simulink model "DDMRModel"  (R2023b)
settings: Solver=VariableStepAuto  StartTime=0.0  StopTime=3  RelTol=1e-3
undefined symbols (not defined in the file or in its folder): Bm, gR, Jm, Kd, ke, Ki, Kp, kt, L, La, R, Ra
settings Model: Creator=rodrigoscott  LastModifiedBy=rodrigoscott

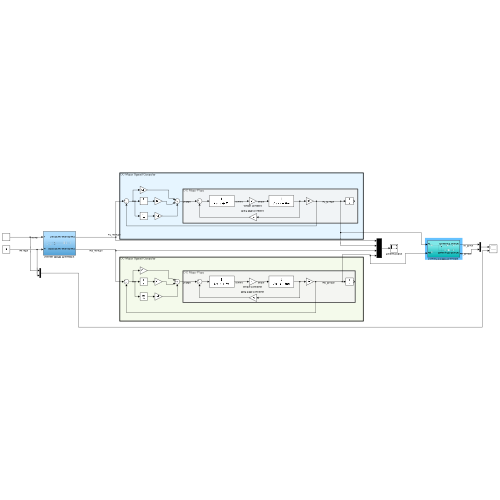
[thumbnail: Simulink's stored preview of the top-level diagram]
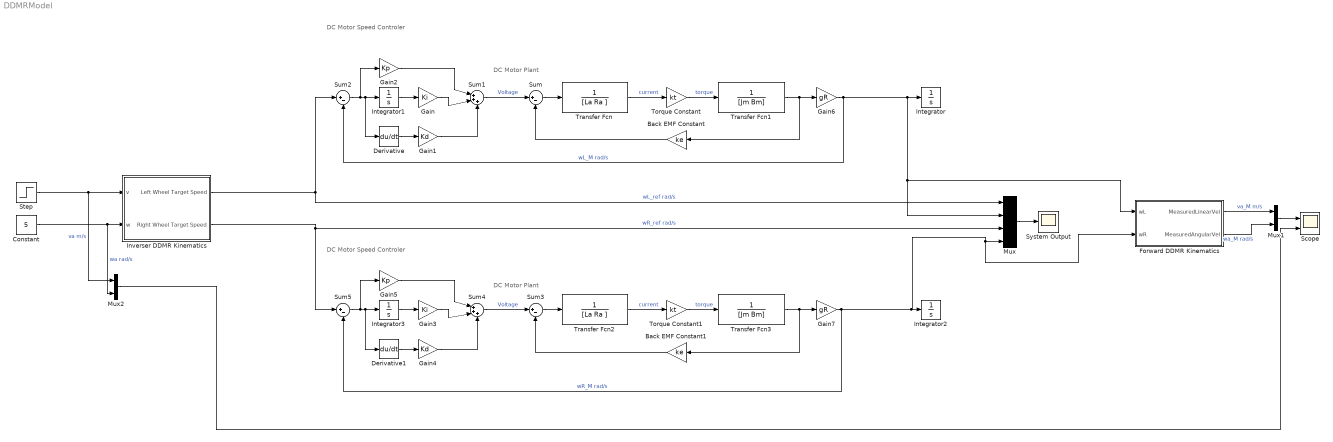
== system DDMRModel ==
  note: DC Motor Speed Controler
  note: DC Motor Plant
  note: DC Motor Plant
  note: DC Motor Speed Controler
  Back EMF Constant : Gain  Gain=ke
  Back EMF Constant1 : Gain  Gain=ke
  Constant : Constant  Value=5
  Derivative : Derivative
  Derivative1 : Derivative
  Forward DDMR Kinematics : Subsystem
  Gain : Gain  Gain=Ki
  Gain1 : Gain  Gain=Kd
  Gain2 : Gain  Gain=Kp
  Gain3 : Gain  Gain=Ki
  Gain4 : Gain  Gain=Kd
  Gain5 : Gain  Gain=Kp
  Gain6 : Gain  Gain=gR
  Gain7 : Gain  Gain=gR
  Integrator{,1..3} (4 alike) : Integrator
  Inverser DDMR Kinematics : Subsystem
  Mux : Mux
  Mux1 : Mux  Inputs=2
  Mux2 : Mux  Inputs=2
  Scope : Scope  NumInputPorts=2
  Step : Step  Time=0  SampleTime=0
  Sum{,2..3,5} (4 alike) : Sum  Inputs=|+-
  Sum1 : Sum  Inputs=|+++
  Sum4 : Sum  Inputs=|+++
  System Output : Scope
  Torque Constant : Gain  Gain=kt
  Torque Constant1 : Gain  Gain=kt
  Transfer Fcn : TransferFcn  Denominator=[La Ra ]
  Transfer Fcn1 : TransferFcn  Denominator=[Jm Bm]
  Transfer Fcn2 : TransferFcn  Denominator=[La Ra ]
  Transfer Fcn3 : TransferFcn  Denominator=[Jm Bm]
  wires:
  Sum1/1 -> Sum/1  "Voltage"
  Transfer Fcn/1 -> Torque Constant/1  "current"
  Sum/1 -> Transfer Fcn/1
  Transfer Fcn1/1 -> Back EMF Constant/1, Gain6/1
  Sum2/1 -> Gain2/1, Derivative/1, Integrator1/1
  Back EMF Constant/1 -> Sum/2
  Gain1/1 -> Sum1/3
  Torque Constant/1 -> Transfer Fcn1/1  "torque"
  Integrator1/1 -> Gain/1
  Gain/1 -> Sum1/2
  Gain2/1 -> Sum1/1
  Derivative/1 -> Gain1/1
  Transfer Fcn3/1 -> Back EMF Constant1/1, Gain7/1
  Back EMF Constant1/1 -> Sum3/2
  Transfer Fcn2/1 -> Torque Constant1/1  "current"
  Torque Constant1/1 -> Transfer Fcn3/1  "torque"
  Gain4/1 -> Sum4/3
  Sum3/1 -> Transfer Fcn2/1
  Sum5/1 -> Gain5/1, Derivative1/1, Integrator3/1
  Gain3/1 -> Sum4/2
  Gain5/1 -> Sum4/1
  Derivative1/1 -> Gain4/1
  Sum4/1 -> Sum3/1  "Voltage"
  Integrator3/1 -> Gain3/1
  Inverser DDMR Kinematics/1(Left Wheel Target Speed) -> Sum2/1, Mux/1  "wL_ref rad/s"
  Inverser DDMR Kinematics/2(Right Wheel Target Speed) -> Sum5/1, Mux/3  "wR_ref rad/s"
  Step/1 -> Mux2/1, Inverser DDMR Kinematics/1(v)  "va m/s"
  Constant/1 -> Mux2/2, Inverser DDMR Kinematics/2(w)  "wa rad/s"
  Gain6/1 -> Sum2/2, Integrator/1, Mux/2, Forward DDMR Kinematics/1(wL)  "wL_M rad/s"
  Gain7/1 -> Integrator2/1, Forward DDMR Kinematics/2(wR), Mux/4, Sum5/2  "wR_M rad/s"
  Mux/1 -> System Output/1
  Forward DDMR Kinematics/1(MeasuredLinearVel) -> Mux1/1  "va_M m/s"
  Forward DDMR Kinematics/2(MeasuredAngularVel) -> Mux1/2  "wa_M rad/s"
  Mux2/1 -> Scope/2
  Mux1/1 -> Scope/1

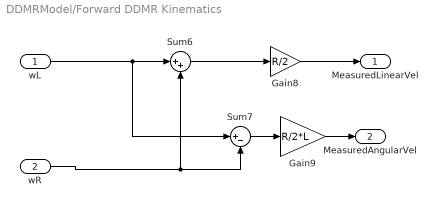
== system DDMRModel/Forward DDMR Kinematics ==
  wL : Inport
  wR : Inport  Port=2
  Gain8 : Gain  Gain=R/2
  Gain9 : Gain  Gain=R/2*L
  Sum6 : Sum  Inputs=|++
  Sum7 : Sum  Inputs=|+-
  MeasuredLinearVel : Outport
  MeasuredAngularVel : Outport  Port=2
  wires:
  Gain8/1 -> MeasuredLinearVel/1
  wR/1 -> Sum7/2, Sum6/2
  Sum7/1 -> Gain9/1
  wL/1 -> Sum7/1, Sum6/1
  Gain9/1 -> MeasuredAngularVel/1
  Sum6/1 -> Gain8/1

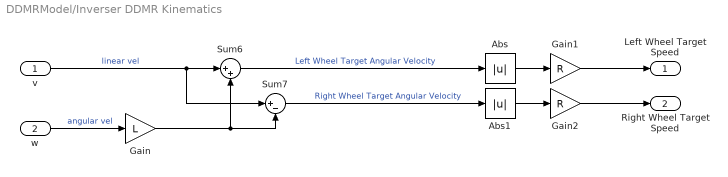
== system DDMRModel/Inverser DDMR Kinematics ==
  v : Inport
  w : Inport  Port=2
  Abs : Abs  SaturateOnIntegerOverflow=off
  Abs1 : Abs  SaturateOnIntegerOverflow=off
  Gain : Gain  Gain=L
  Gain1 : Gain  Gain=R
  Gain2 : Gain  Gain=R
  Sum6 : Sum  Inputs=|++
  Sum7 : Sum  Inputs=|+-
  Left Wheel Target Speed : Outport
  Right Wheel Target Speed : Outport  Port=2
  wires:
  v/1 -> Sum7/1, Sum6/1  "linear vel"
  Sum7/1 -> Abs1/1  "Right Wheel Target Angular Velocity"
  w/1 -> Gain/1  "angular vel"
  Sum6/1 -> Abs/1  "Left Wheel Target Angular Velocity"
  Gain/1 -> Sum7/2, Sum6/2
  Abs/1 -> Gain1/1
  Abs1/1 -> Gain2/1
  Gain1/1 -> Left Wheel Target Speed/1
  Gain2/1 -> Right Wheel Target Speed/1
